simulink model "Calculating_Distance"  (R2021a)
settings: Solver=VariableStepAuto  StartTime=0.0  StopTime=10.0  RelTol=1e-3
settings Model: Creator=HP  LastModifiedBy=HP

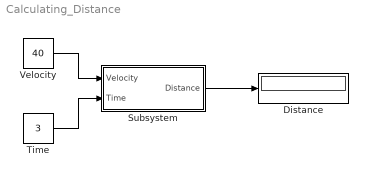
== system Calculating_Distance ==
  Distance : Display
  Subsystem : Subsystem
  Time : Constant  Value=3
  Velocity : Constant  Value=40
  wires:
  Subsystem/1(Distance) -> Distance/1
  Time/1 -> Subsystem/2(Time)
  Velocity/1 -> Subsystem/1(Velocity)

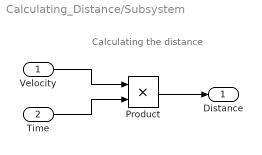
== system Calculating_Distance/Subsystem ==
  note: Calculating the distance
  Velocity : Inport
  Time : Inport  Port=2
  Product : Product
  Distance : Outport
  wires:
  Product/1 -> Distance/1
  Time/1 -> Product/2
  Velocity/1 -> Product/1
